simulink model "chaos_ofdm_model_tx_rx"  (R2015b)
settings: Solver=VariableStepDiscrete  SolverMode=SingleTasking  StartTime=0.0  StopTime=inf  RelTol=1e-3
libraries: dspxfrm3 x2, commdigbbndam3 x2, simulink_extras x1, dspsrcs4 x1
settings Model: Creator=bam-bam81  LastModifiedBy=bam-bam81
settings DataIOCC: SaveFormat=Array  SaveOutput=off  SaveTime=off
settings OptimizationCC: BooleanDataType=off  DefaultParameterBehavior=Inlined  LocalBlockOutputs=off
settings DebuggingCC: AlgebraicLoopMsg=error  SolverPrmCheckMsg=warning  SingleTaskRateTransMsg=error
settings GRTTargetCC: GeneratePreprocessorConditionals=Disable all
settings ConfigComp: CovModelRefEnable=Off  CovSFcnEnable=off

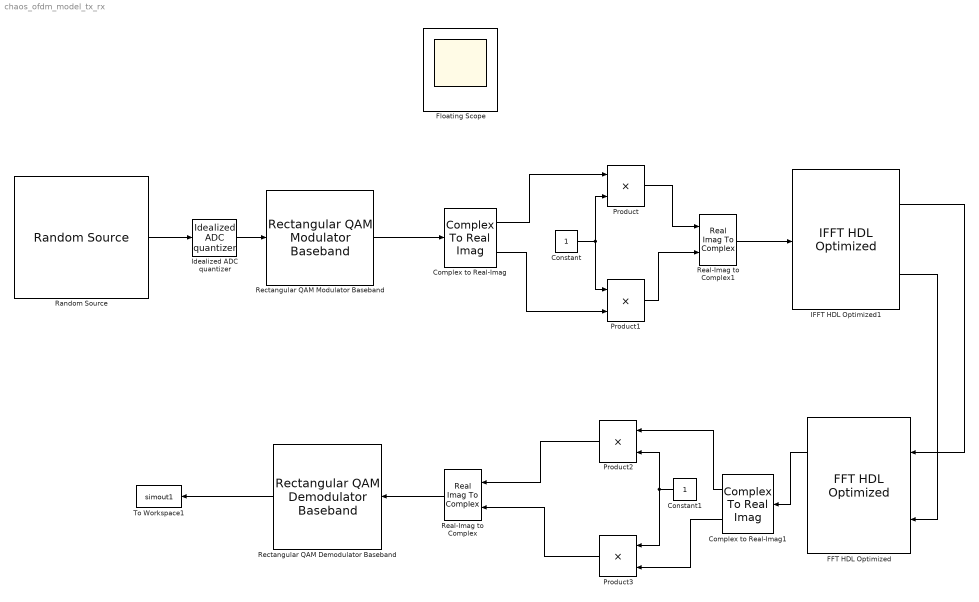
== system chaos_ofdm_model_tx_rx ==
  Complex to Real-Imag : ComplexToRealImag
  Complex to Real-Imag1 : ComplexToRealImag
  Constant : Constant  SampleTime=-1
  Constant1 : Constant  SampleTime=-1
  FFT HDL Optimized : dspxfrm3/FFT HDL Optimized  BitReversedOutput=on  Normalize=off  FFTLengthSource=Property  FFTLength=256  RoundingMethod=Floor  OverflowAction=Wrap  ValidInputPort=on  ResetInputPort=off  StartOutputPort=off  EndOutputPort=off  SimulateUsing=Code generation
  Floating Scope : Scope
      settings: Floating=on
  IFFT HDL Optimized1 : dspxfrm3/IFFT HDL Optimized  BitReversedOutput=on  Normalize=on  FFTLengthSource=Property  FFTLength=256  RoundingMethod=Floor  OverflowAction=Wrap  ValidInputPort=off  ResetInputPort=off  StartOutputPort=off  EndOutputPort=off  SimulateUsing=Code generation
  Idealized ADC quantizer : simulink_extras/Additional Discrete/Idealized ADC quantizer  NumberOfConverterBits=4  Vmin=0  Vmax=5  OutputDataType=int16  OutputNegativeValues=off
  Product : Product  InputSameDT=on
  Product1 : Product  InputSameDT=on
  Product2 : Product  OutDataTypeStr=Inherit: Inherit via back propagation
  Product3 : Product  OutDataTypeStr=Inherit: Inherit via back propagation
  Random Source : dspsrcs4/Random Source  SrcType=Gaussian  NormMethod=Ziggurat  CltLength=12  MinVal=0  MaxVal=1  MeanVal=0  VarVal=1  RepMode=Not repeatable  rawSeed=1  IsInherit=off  SampMode=Discrete  SampTime=1  SampFrame=1  DataType=Single  OutComplex=Real  OutputFrames=off
  Real-Imag to Complex : RealImagToComplex
  Real-Imag to Complex1 : RealImagToComplex
  Rectangular QAM Demodulator Baseband : commdigbbndam3/Rectangular QAM Demodulator Baseband  M=4  PowType=Min. distance between symbols  MinDist=2  AvgPow=1  PeakPow=1  Ph=0  Dec=Gray  Mapping=[0:15]  OutType=Integer  DecType=Hard decision  VarSource=Dialog  Variance=1  outDtype1=Inherit via internal rule  outDtype2=Inherit via internal rule  derotateFactorWordLen=16  denormFactorWordLen=16  prodOutWordLen=32  prodOutRoundingMode=Floor  prodOutOverflowMode=Wrap  sumWordLen=32
  Rectangular QAM Modulator Baseband : commdigbbndam3/Rectangular QAM Modulator Baseband  M=16  InType=Integer  Enc=Gray  Mapping=[0:15]  PowType=Min. distance between symbols  MinDist=2  AvgPow=1  PeakPow=1  Ph=0  outDtype=double  outWordLen=16  outUDDataType=sfix(16)  outFracLenMode=Best precision  outFracLen=15
  To Workspace1 : ToWorkspace  VariableName=simout1  SaveFormat=Timeseries  SampleTime=-1
  wires:
  Rectangular QAM Modulator Baseband/1 -> Complex to Real-Imag/1
  Real-Imag to Complex1/1 -> IFFT HDL Optimized1/1
  Product/1 -> Real-Imag to Complex1/1
  Product1/1 -> Real-Imag to Complex1/2
  Complex to Real-Imag/1 -> Product/1
  Complex to Real-Imag/2 -> Product1/2
  Constant/1 -> Product1/1, Product/2
  Product2/1 -> Real-Imag to Complex/1
  Product3/1 -> Real-Imag to Complex/2
  Constant1/1 -> Product3/1, Product2/2
  FFT HDL Optimized/1 -> Complex to Real-Imag1/1
  IFFT HDL Optimized1/1 -> FFT HDL Optimized/1
  IFFT HDL Optimized1/2 -> FFT HDL Optimized/2
  Complex to Real-Imag1/1 -> Product2/1
  Complex to Real-Imag1/2 -> Product3/2
  Random Source/1 -> Idealized ADC quantizer/1
  Rectangular QAM Demodulator Baseband/1 -> To Workspace1/1
  Real-Imag to Complex/1 -> Rectangular QAM Demodulator Baseband/1
  Idealized ADC quantizer/1 -> Rectangular QAM Modulator Baseband/1
